simulink model "drive4"  (R2015a)
settings: Solver=ode45  StartTime=0.0  StopTime=5  MaxStep=dt  RelTol=1e-5  AbsTol=1e-4
undefined symbols (not defined in the file or in its folder): bcin, bcout, Bd, Bt, dt, Gbx, init_angvel, Itime, Itorq, Je, Jt, Jv, Jw, kcin, kcout, Kd, L
settings Model: ExtModeTrigMode=oneshot  ExtModeArmWhenConnect=off  Creator=ttmcb  LastModifiedBy=ttmcb
settings DataIOCC: LimitDataPoints=off  SignalLoggingSaveFormat=ModelDataLogs  SaveOutput=off  SaveTime=off  SignalLoggingName=sigsOut
settings OptimizationCC: BooleanDataType=off  ExpressionDepthLimit=2147483647  InitFltsAndDblsToZero=on
settings DebuggingCC: SaveWithParameterizedLinksMsg=none  UnderspecifiedInitializationDetection=Classic  MergeDetectMultiDrivingBlocksExec=none  SignalResolutionControl=TryResolveAllWithWarning  MultiTaskDSMMsg=warning  MultiTaskCondExecSysMsg=none  FcnCallInpInsideContextMsg=UseLocalSettings  StateNameClashWarn=warning  StrictBusMsg=None
settings HardwareCC: TargetUnknown=on
settings GRTTargetCC: TargetFcnLib=ansi_tfl_tmw.mat  CombineOutputUpdateFcns=off  GRTInterface=on

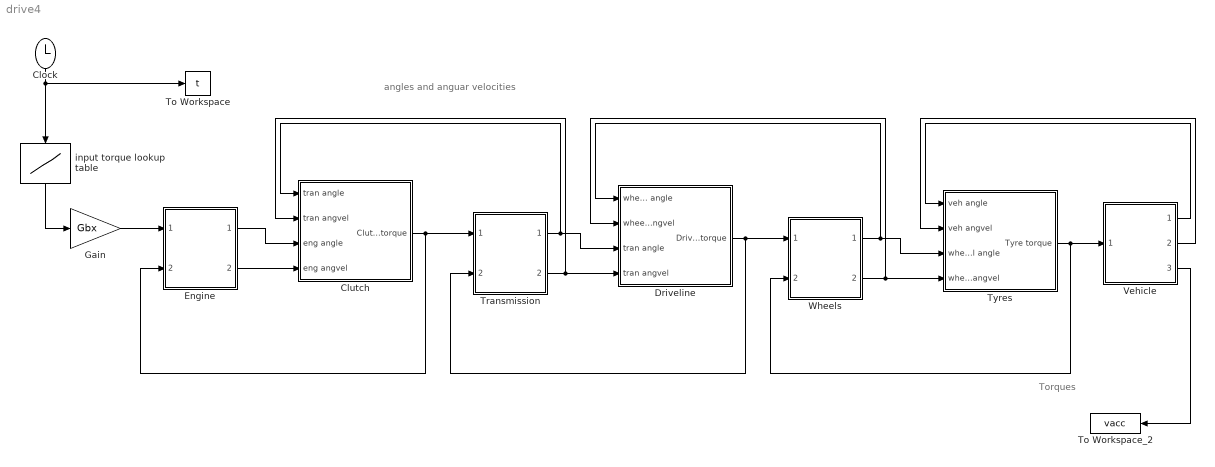
== system drive4 ==
  note: angles and
      | anguar velocities
  note: Torques
  Clock : Clock
  Clutch : Subsystem
      mask Display: plot([-1,-1],[1,9],[25,25],[1,9],[-1,3,[4:2:20],21,25],[7,7,8,6,8,6,8,6,8,6,8,7,7],[-1,3,3,21],[3,3,4,4],[3,3,21],[3,2,2],[13,13],[3.8,2.2],[13,25],[3,3])
  Driveline : Subsystem
      mask Display: plot([-1,-1],[1,9],[25,25],[1,9],[-1,3,[4:2:20],21,25],[7,7,8,6,8,6,8,6,8,6,8,7,7],[-1,3,3,21],[3,3,4,4],[3,3,21],[3,2,2],[13,13],[3.8,2.2],[13,25],[3,3])
  Engine : Subsystem
      mask Display: disp('Je')
  Gain : Gain  Gain=Gbx  SaturateOnIntegerOverflow=on  OutDataTypeStr=Inherit: Same as input  ParamDataTypeStr=Inherit: Same as input
  To Workspace : ToWorkspace  VariableName=t  SampleTime=dt
      settings: MaxDataPoints=1e5
  To Workspace_2 : ToWorkspace  VariableName=vacc  SampleTime=dt
      settings: MaxDataPoints=1e5
  Transmission : Subsystem
      mask Display: disp('Jt')
  Tyres : Subsystem
      mask Display: plot([-1,-1],[1,5],[25,25],[1,5],[-1,3,3,21],[3,3,4,4],[3,3,21],[3,2,2],[13,13],[3.8,2.2],[13,25],[3,3])
  Vehicle : Subsystem
      mask Display: disp('Jv')
  Wheels : Subsystem
      mask Display: disp('Jw')
  input torque lookup table : Lookup  InputValues=Itime  Table=Itorq  SaturateOnIntegerOverflow=on
  wires:
  Vehicle/2(veh angvel) -> Tyres/2(veh angvel)
  Vehicle/1(veh angle) -> Tyres/1(veh angle)
  Wheels/2(wheel angvel) -> Tyres/4(wheel angvel), Driveline/2(wheel angvel)
  Wheels/1(wheel angle) -> Tyres/3(wheel angle), Driveline/1(wheel angle)
  Tyres/1(Tyre torque) -> Vehicle/1(Tyre torque), Wheels/2(Tyre torque)
  Transmission/2(tran angvel) -> Driveline/4(tran angvel), Clutch/2(tran angvel)
  Transmission/1(tran angle) -> Driveline/3(tran angle), Clutch/1(tran angle)
  Engine/1(eng angle) -> Clutch/3(eng angle)
  Engine/2(eng angvel) -> Clutch/4(eng angvel)
  Driveline/1(Driveline torque) -> Wheels/1(Driveline torque), Transmission/2(Driveline torque)
  Clutch/1(Clutch torque) -> Transmission/1(Clutch torque), Engine/2(Clutch torque)
  Clock/1 -> To Workspace/1, input torque lookup table/1
  Vehicle/3(veh angacc) -> To Workspace_2/1
  input torque lookup table/1 -> Gain/1
  Gain/1 -> Engine/1(Input torque)

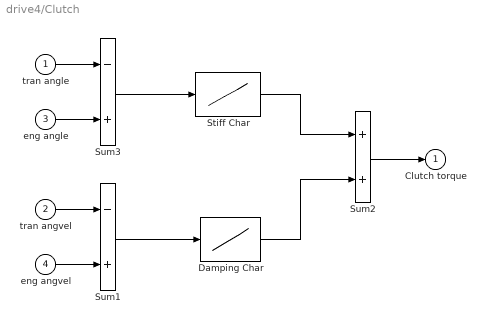
== system drive4/Clutch ==
  tran angle : Inport
  tran angvel : Inport  Port=2
  eng angle : Inport  Port=3
  eng angvel : Inport  Port=4
  Damping Char : Lookup  InputValues=bcin  Table=bcout  SaturateOnIntegerOverflow=on
  Stiff Char : Lookup  InputValues=kcin  Table=kcout  SaturateOnIntegerOverflow=on
  Sum1 : Sum  Inputs=-+  SaturateOnIntegerOverflow=on  InputSameDT=on  OutDataTypeStr=Inherit: Same as first input
  Sum2 : Sum  SaturateOnIntegerOverflow=on  InputSameDT=on  OutDataTypeStr=Inherit: Same as first input
  Sum3 : Sum  Inputs=-+  SaturateOnIntegerOverflow=on  InputSameDT=on  OutDataTypeStr=Inherit: Same as first input
  Clutch torque : Outport
  wires:
  eng angvel/1 -> Sum1/2
  tran angvel/1 -> Sum1/1
  Sum2/1 -> Clutch torque/1
  eng angle/1 -> Sum3/2
  tran angle/1 -> Sum3/1
  Sum1/1 -> Damping Char/1
  Sum3/1 -> Stiff Char/1
  Stiff Char/1 -> Sum2/1
  Damping Char/1 -> Sum2/2

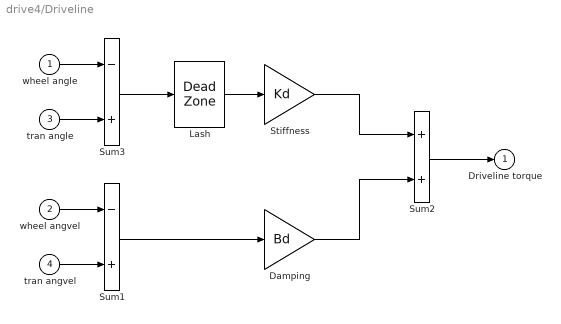
== system drive4/Driveline ==
  wheel angle : Inport
  wheel angvel : Inport  Port=2
  tran angle : Inport  Port=3
  tran angvel : Inport  Port=4
  "Damping " : Gain  Gain=Bd  SaturateOnIntegerOverflow=on  OutDataTypeStr=Inherit: Same as input  ParamDataTypeStr=Inherit: Same as input
  Lash : DeadZone  LowerValue=-0.5*L  UpperValue=0.5*L  SaturateOnIntegerOverflow=on
  Stiffness : Gain  Gain=Kd  SaturateOnIntegerOverflow=on  OutDataTypeStr=Inherit: Same as input  ParamDataTypeStr=Inherit: Same as input
  Sum1 : Sum  Inputs=-+  SaturateOnIntegerOverflow=on  InputSameDT=on  OutDataTypeStr=Inherit: Same as first input
  Sum2 : Sum  SaturateOnIntegerOverflow=on  InputSameDT=on  OutDataTypeStr=Inherit: Same as first input
  Sum3 : Sum  Inputs=-+  SaturateOnIntegerOverflow=on  InputSameDT=on  OutDataTypeStr=Inherit: Same as first input
  Driveline torque : Outport
  wires:
  "Damping "/1 -> Sum2/2
  Stiffness/1 -> Sum2/1
  Sum1/1 -> "Damping "/1
  wheel angle/1 -> Sum3/1
  tran angle/1 -> Sum3/2
  Sum2/1 -> Driveline torque/1
  wheel angvel/1 -> Sum1/1
  tran angvel/1 -> Sum1/2
  Sum3/1 -> Lash/1
  Lash/1 -> Stiffness/1

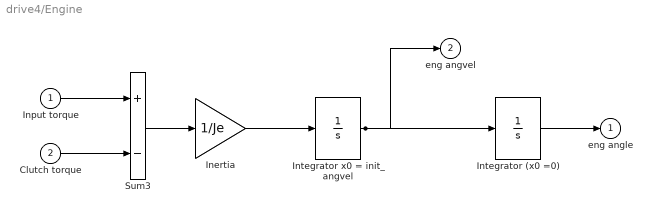
== system drive4/Engine ==
  Input torque : Inport
  Clutch torque : Inport  Port=2
  Inertia : Gain  Gain=1/Je  SaturateOnIntegerOverflow=on  OutDataTypeStr=Inherit: Same as input  ParamDataTypeStr=Inherit: Same as input
  Integrator (x0 =0) : Integrator
  Integrator x0 = init_angvel : Integrator  InitialCondition=init_angvel
  Sum3 : Sum  Inputs=+-  SaturateOnIntegerOverflow=on  InputSameDT=on  OutDataTypeStr=Inherit: Same as first input
  eng angle : Outport
  eng angvel : Outport  Port=2
  wires:
  Integrator (x0 =0)/1 -> eng angle/1
  Integrator x0 = init_angvel/1 -> eng angvel/1, Integrator (x0 =0)/1
  Inertia/1 -> Integrator x0 = init_angvel/1
  Sum3/1 -> Inertia/1
  Input torque/1 -> Sum3/1
  Clutch torque/1 -> Sum3/2

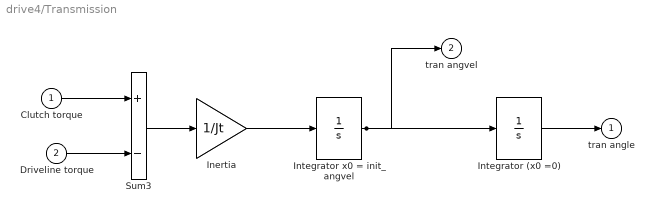
== system drive4/Transmission ==
  Clutch torque : Inport
  Driveline torque : Inport  Port=2
  Inertia : Gain  Gain=1/Jt  SaturateOnIntegerOverflow=on  OutDataTypeStr=Inherit: Same as input  ParamDataTypeStr=Inherit: Same as input
  Integrator (x0 =0) : Integrator
  Integrator x0 = init_angvel : Integrator  InitialCondition=init_angvel
  Sum3 : Sum  Inputs=+-  SaturateOnIntegerOverflow=on  InputSameDT=on  OutDataTypeStr=Inherit: Same as first input
  tran angle : Outport
  tran angvel : Outport  Port=2
  wires:
  Driveline torque/1 -> Sum3/2
  Clutch torque/1 -> Sum3/1
  Sum3/1 -> Inertia/1
  Inertia/1 -> Integrator x0 = init_angvel/1
  Integrator (x0 =0)/1 -> tran angle/1
  Integrator x0 = init_angvel/1 -> Integrator (x0 =0)/1, tran angvel/1

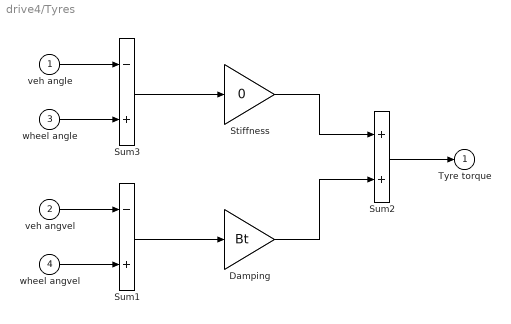
== system drive4/Tyres ==
  veh angle : Inport
  veh angvel : Inport  Port=2
  wheel angle : Inport  Port=3
  wheel angvel : Inport  Port=4
  "Damping " : Gain  Gain=Bt  SaturateOnIntegerOverflow=on  OutDataTypeStr=Inherit: Same as input  ParamDataTypeStr=Inherit: Same as input
  Stiffness : Gain  Gain=0  SaturateOnIntegerOverflow=on  OutDataTypeStr=Inherit: Same as input  ParamDataTypeStr=Inherit: Same as input
  Sum1 : Sum  Inputs=-+  SaturateOnIntegerOverflow=on  InputSameDT=on  OutDataTypeStr=Inherit: Same as first input
  Sum2 : Sum  SaturateOnIntegerOverflow=on  InputSameDT=on  OutDataTypeStr=Inherit: Same as first input
  Sum3 : Sum  Inputs=-+  SaturateOnIntegerOverflow=on  InputSameDT=on  OutDataTypeStr=Inherit: Same as first input
  Tyre torque : Outport
  wires:
  "Damping "/1 -> Sum2/2
  Stiffness/1 -> Sum2/1
  Sum3/1 -> Stiffness/1
  Sum1/1 -> "Damping "/1
  veh angle/1 -> Sum3/1
  wheel angle/1 -> Sum3/2
  Sum2/1 -> Tyre torque/1
  veh angvel/1 -> Sum1/1
  wheel angvel/1 -> Sum1/2

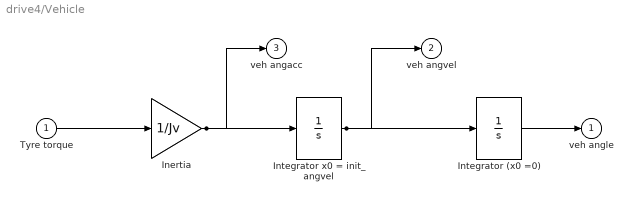
== system drive4/Vehicle ==
  Tyre torque : Inport
  Inertia : Gain  Gain=1/Jv  SaturateOnIntegerOverflow=on  OutDataTypeStr=Inherit: Same as input  ParamDataTypeStr=Inherit: Same as input
  Integrator (x0 =0) : Integrator
  Integrator x0 = init_angvel : Integrator  InitialCondition=init_angvel
  veh angle : Outport
  veh angvel : Outport  Port=2
  veh angacc : Outport  Port=3
  wires:
  Integrator (x0 =0)/1 -> veh angle/1
  Integrator x0 = init_angvel/1 -> veh angvel/1, Integrator (x0 =0)/1
  Tyre torque/1 -> Inertia/1
  Inertia/1 -> Integrator x0 = init_angvel/1, veh angacc/1

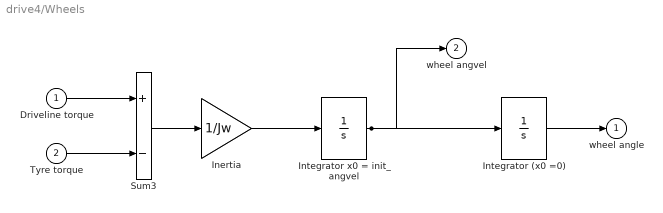
== system drive4/Wheels ==
  Driveline torque : Inport
  Tyre torque : Inport  Port=2
  Inertia : Gain  Gain=1/Jw  SaturateOnIntegerOverflow=on  OutDataTypeStr=Inherit: Same as input  ParamDataTypeStr=Inherit: Same as input
  Integrator (x0 =0) : Integrator
  Integrator x0 = init_angvel : Integrator  InitialCondition=init_angvel
  Sum3 : Sum  Inputs=+-  SaturateOnIntegerOverflow=on  InputSameDT=on  OutDataTypeStr=Inherit: Same as first input
  wheel angle : Outport
  wheel angvel : Outport  Port=2
  wires:
  Tyre torque/1 -> Sum3/2
  Driveline torque/1 -> Sum3/1
  Sum3/1 -> Inertia/1
  Inertia/1 -> Integrator x0 = init_angvel/1
  Integrator (x0 =0)/1 -> wheel angle/1
  Integrator x0 = init_angvel/1 -> Integrator (x0 =0)/1, wheel angvel/1
